simulink model "Tank2_Primitives"  (R2012b)
settings: Solver=FixedStepDiscrete  StartTime=0.0  StopTime=10.0  FixedStep=0.1  RelTol=1e-3
libraries: simulink x1
settings Model: Creator=Kerianne  LastModifiedBy=Kerianne
settings DataIOCC: SaveFormat=Structure
settings OptimizationCC: InlineParams=on

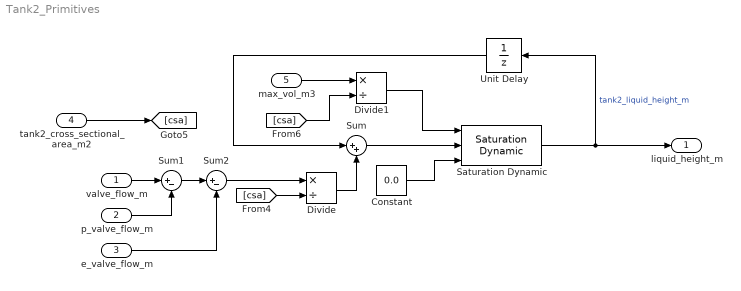
== system Tank2_Primitives ==
  valve_flow_m : Inport
  p_valve_flow_m : Inport  Port=2
  e_valve_flow_m : Inport  Port=3
  tank2_cross_sectional_area_m2 : Inport  Port=4
  max_vol_m3 : Inport  Port=5
  Constant : Constant  Value=0.0
  Divide : Product  Inputs=*/
  Divide1 : Product  Inputs=*/
  Saturation Dynamic : simulink/Discontinuities/Saturation Dynamic  OutMin=[]  OutMax=[]  OutDataTypeStr=Inherit: Same as second input  OutDataType=fixdt(1, 16)  OutScaling=2^-10  DoSatur=off
  Sum : Sum  Inputs=|++
  Sum1 : Sum  Inputs=|+-
  Sum2 : Sum  Inputs=|+-
  Unit Delay : UnitDelay  SampleTime=-1
  liquid_height_m : Outport
  wires:
  valve_flow_m/1 -> Sum1/1
  p_valve_flow_m/1 -> Sum1/2
  Divide/1 -> Sum/2
  [csa] -> Divide/2
  tank2_cross_sectional_area_m2/1 -> [csa]
  e_valve_flow_m/1 -> Sum2/2
  Sum2/1 -> Divide/1
  Sum1/1 -> Sum2/1
  max_vol_m3/1 -> Divide1/1
  Divide1/1 -> Saturation Dynamic/1
  Sum/1 -> Saturation Dynamic/2
  Constant/1 -> Saturation Dynamic/3
  [csa] -> Divide1/2
  Saturation Dynamic/1 -> Unit Delay/1, liquid_height_m/1  "tank2_liquid_height_m"
  Unit Delay/1 -> Sum/1
